simulink model "TD2_L_MODEL"  (Simulink 7.6)
settings: Solver=ode45  StartTime=0.0  StopTime=10  RelTol=1e-3
libraries: simulink x1
settings Model: Creator=Administrator  LastModifiedBy=Administrator
settings DebuggingCC: SolverPrmCheckMsg=none

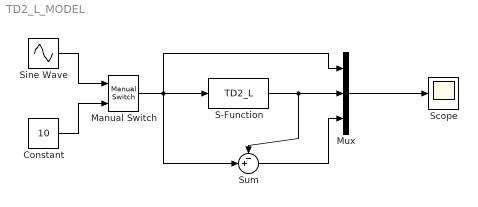
== system TD2_L_MODEL ==
  Constant : Constant  Value=10  SampleTime=0.01
  Manual Switch : simulink/Signal Routing/Manual Switch  SystemSampleTime=-1  sw=0  action=0  varsize=off
  Mux : Mux  Inputs=3
  S-Function : S-Function  FunctionName=TD2_L  Parameters=r,h  EnableBusSupport=off  mask{r=5, h=0.01}
      mask prompts: r "r="; h "h="
  Scope : Scope
      settings: TimeRange=5  YMin=0  YMax=10
  Sine Wave : Sin  Frequency=pi/2  SampleTime=0
  Sum : Sum  Inputs=-+|
  wires:
  Manual Switch/1 -> Mux/1, Sum/2, S-Function/1
  Mux/1 -> Scope/1
  S-Function/1 -> Mux/2, Sum/1
  Sine Wave/1 -> Manual Switch/1
  Constant/1 -> Manual Switch/2
  Sum/1 -> Mux/3
